simulink model "robo"  (R2024b)
settings: Solver=ode45  StartTime=0.0  StopTime=inf  FixedStep=0.050  RelTol=1e-3
model workspace (MAT data in the model file):
  Sig = Simulink.Signal
  Sig.Dimensions = -1
  Sig.DimensionsMode = 'auto'
  Sig.Complexity = 'auto'
  Sig.SampleTime = -1
  Sig.SamplingMode = 'auto'
  Sig.DataType = 'auto'
  Var = 0
libraries: fuzblock x2
settings Model: PauseTimes=7  Creator=user  LastModifiedBy=manav
settings SolverCC: AlgebraicLoopSolver=TrustRegion
settings DataIOCC: LimitDataPoints=on  SaveFormat=Array  ReturnWorkspaceOutputs=off
settings OptimizationCC: BlockReduction=off  BooleanDataType=off  LifeSpan=inf
settings DebuggingCC: SaveWithParameterizedLinksMsg=none  UnderspecifiedInitializationDetection=Classic  MergeDetectMultiDrivingBlocksExec=none  SignalResolutionControl=TryResolveAllWithWarning  UnconnectedInputMsg=warning  UnconnectedOutputMsg=warning  UnconnectedLineMsg=warning  SFUnexpectedBacktrackingDiag=warning  SFNoUnconditionalDefaultTransitionDiag=warning  SFExecutionAtInitializationDiag=none  ArithmeticOperatorsInVariantConditions=warning
settings HardwareCC: ProdBitPerPointer=32  ProdBitPerSizeT=32  ProdBitPerPtrDiffT=32  ProdLargestAtomicFloat=None  ProdIntDivRoundTo=Undefined  ProdEndianess=Unspecified  ProdWordSize=32  ProdHWDeviceType=32-bit Generic  TargetUnknown=on
settings ModelReferenceCC: EnableRefExpFcnMdlSchedulingChecks=on  PropagateSignalLabelsOutOfModel=off
settings SFSimCC: SimUseLocalCustomCode=off  CustomCodeUndefinedFunction=UseInterfaceOnly
settings RTWCC: RTWUseLocalCustomCode=off  GPUComputeCapability=3.5
settings CodeAppCC: StateflowObjectComments=on
settings GRTTargetCC: TargetLangStandard=C89/C90 (ANSI)
settings ConfigComp: CovMetricSettings=dw  CovSaveCumulativeToWorkspaceVar=on  CovSaveSingleToWorkspaceVar=on  CovExternalEMLEnable=off  CovSFcnEnable=off

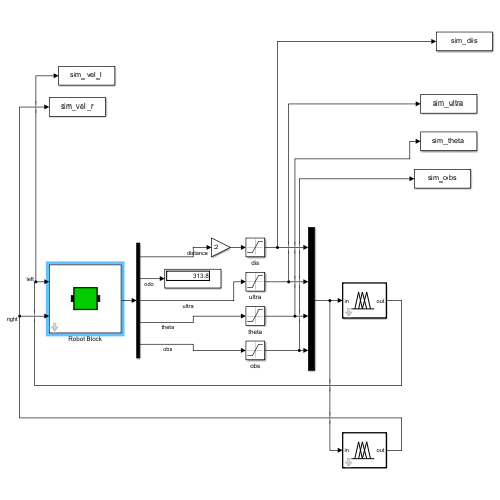
[thumbnail: Simulink's stored preview of the top-level diagram]
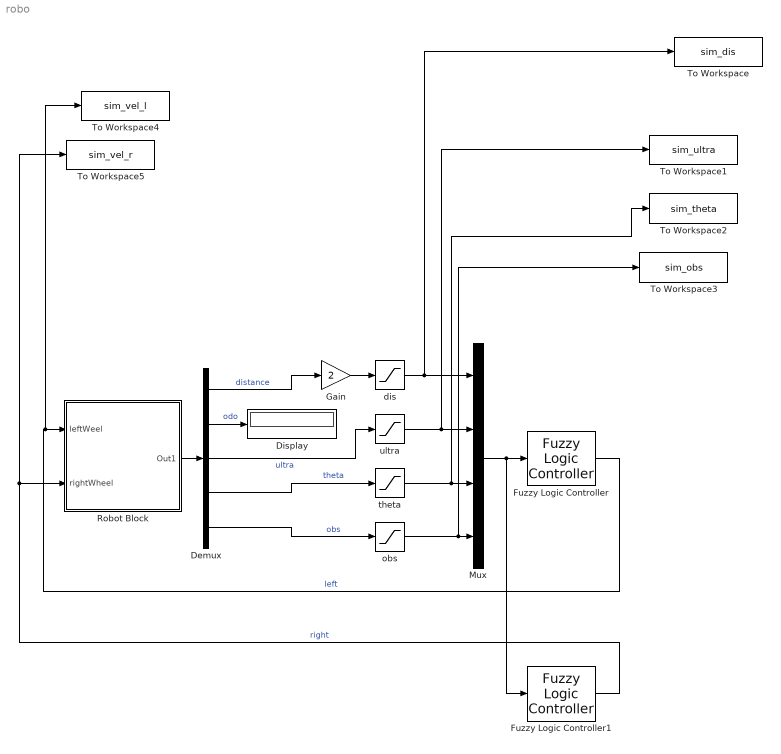
== system robo ==
  Demux : Demux  Outputs=5
  Display : Display
  Fuzzy Logic Controller : fuzblock/Fuzzy Logic  Controller  FIS='anfis_l.fis'  OutputSampleNumber=101  DataType=double  FuzzifiedInputs=off  RuleFiringStrengths=off  RuleOutputs=off  AggregatedOutputs=off  SimulateUsing=Interpreted execution  OutOfRangeInputValueMessage=warning  NoRuleFiredMessage=warning  EmptyOutputFuzzySetMessage=warning
  Fuzzy Logic Controller1 : fuzblock/Fuzzy Logic  Controller  FIS='anfis_r.fis'  OutputSampleNumber=101  DataType=double  FuzzifiedInputs=off  RuleFiringStrengths=off  RuleOutputs=off  AggregatedOutputs=off  SimulateUsing=Interpreted execution  OutOfRangeInputValueMessage=warning  NoRuleFiredMessage=warning  EmptyOutputFuzzySetMessage=warning
  Gain : Gain  Gain=2
  Mux : Mux
  Robot Block : Subsystem  mask(Two-wheel Mobile Robot Model){stID=8199607, modeVal=off, initAngle=1.696, simStep=0.050, Xpos=3.4, Ypos=5.8, isDemo=off}
      mask prompts: stID "Please Enter your UOW student number"; modeVal "Velocity Measurement Mode, select this to disable animations and to allow for the measurement of the velocity of the robot"; initAngle "Set the starting angle (Radians)"; simStep "Override Simulation Step (Defualt is 0.01)"; Xpos "(X,Y)"
      mask help:
      | Robot: Two-wheel robot is driven by two parallel wheels; the speed of each wheel could be set separately
      | Target: target is a single moving point in 2D space
      | Obstacle: obstacle is a group of polygons.
      | Block inputs:
      | vl : velocity of left wheel
      | vr : velocity of right wheel
      | Range of vl, vr: [-2, 2]
      | Block outputs:
      | theta: angle between robot facing and target bearing
      | dis: distance between robot and target
      | ob_loc
      | Range of obstacle detection sensor is 2.5
      | ob_loc=-9	No obstacle detected
      | ob_loc=-2.5	obstacle detected on the front left
      | ob_loc=-5	obstacle detected on the side left
      | ob_loc=0	obstacle detected in the middle
      | ob_loc=2.5	obstacle detected on the front right
      | ob_loc=5	obstacle detected on the side right
      | Battery level/Odometer: total remaining energy/Distance Travelled
      | ultrasonic: a logorithmic signal indicating the distance to the obstacle ( ie 0 = out of sight , a larger number = nearer to the obstacle )
      |
      | The system will crash if the robot collides with the obstacle.
      mask init:
      | stObj.stID = stID;
      | stObj.modeVal = modeVal;
      | stObj.simStep = simStep;
      | stObj.initPos = [Xpos Ypos initAngle];
      | stObj.isDemo = isDemo;
      mask Help:
      | Robot: Two-wheel robot is driven by two parallel wheels; the speed of each wheel could be set separately
      | Target: target is a single moving point in 2D space
      | Obstacle: obstacle is a group of polygons.
      | Block inputs:
      | vl : velocity of left wheel
      | vr : velocity of right wheel
      | Range of vl, vr: [-2, 2]
      | Block outputs:
      | theta: angle between robot facing and target bearing
      | dis: distance between robot and target
      | ob_loc
      | Range of obstacle detection sensor is 2.5
      | ob_loc=-9	No obstacle detected
      | ob_loc=-2.5	obstacle detected on the front left
      | ob_loc=-5	obstacle detected on the side left
      | ob_loc=0	obstacle detected in the middle
      | ob_loc=2.5	obstacle detected on the front right
      | ob_loc=5	obstacle detected on the side right
      | Battery level/Odometer: total remaining energy/Distance Travelled
      | ultrasonic: a logorithmic signal indicating the distance to the obstacle ( ie 0 = out of sight , a larger number = nearer to the obstacle )
      | 
      | The system will crash if the robot collides with the obstacle.
      mask Callback simStep:
      | pm = Simulink.Mask.get(gcb);
      | simStep = pm.getParameter('simStep');
      | set_param(gcs,'FixedStep', simStep.Value);
      mask DialogControl Container4 Prompt: Set the initial starting Coordinates and angle
      mask DialogControl Control3 Prompt: Set starting Position , (must be in the red shaded region)
      mask DialogControl Control3 Callback:
      | [out,~,~,~,~] = roboanimate_org([],[],[],'setup',[]);
      | Xpos = out(1);
      | Ypos = out(2);
      | p = Simulink.Mask.get(gcb);
      | p.Parameters(1,5).set('Value',num2str(Xpos));
      | p.Parameters(1,6).set('Value',num2str(Ypos));
      mask DialogControl Control5 Prompt: Initial Position:
      mask DialogControl Container4_copy Prompt: Run a demo
      mask DialogControl Control2 Prompt: Run  demo
      mask DialogControl Control2 Callback:
      | if(get_param(gcs,'SimulationStatus') == 'stopped')
      | 
      | pm = Simulink.Mask.get(gcb);
      | pm.Parameters(1,7).set('Value','on');
      | options = simset('SrcWorkspace','current');
      | try
      | sim(gcs,[],options)
      | pm.Parameters(1,7).set('Value','off');
      | catch
      | pm.Parameters(1,7).set('Value','off');
      | end
      | 
      | end
      mask Display:
      | patch([ -0.5 0.5 0.5 -0.5],[ -0.5 -0.5 0.5 0.5],[1 1 1])
      | 
      | patch([ -0.2 0.2 0.2 -0.2],[ -0.05 -0.05 0.05 0.05],[0 0 0])
      | 
      | patch(1.1*[ -0.15  0.15 0.15 -0.15],1.1*[ -0.15 -0.15 0.15 0.15],[0 0 0])
      | 
      | patch([ -0.15  0.15 0.15 -0.15],[ -0.15 -0.15 0.15 0.15],[0 0.8 0])
  To Workspace : ToWorkspace  VariableName=sim_dis  SaveFormat=Timeseries  SampleTime=-1
  To Workspace1 : ToWorkspace  VariableName=sim_ultra  SaveFormat=Timeseries  SampleTime=-1
  To Workspace2 : ToWorkspace  VariableName=sim_theta  SaveFormat=Timeseries  SampleTime=-1
  To Workspace3 : ToWorkspace  VariableName=sim_obs  SaveFormat=Timeseries  SampleTime=-1
  To Workspace4 : ToWorkspace  VariableName=sim_vel_l  SaveFormat=Timeseries  SampleTime=-1
  To Workspace5 : ToWorkspace  VariableName=sim_vel_r  SaveFormat=Timeseries  SampleTime=-1
  dis : Saturate  UpperLimit=20  LowerLimit=0
  obs : Saturate  UpperLimit=5  LowerLimit=-9
  theta : Saturate  UpperLimit=180  LowerLimit=-180
  ultra : Saturate  UpperLimit=25  LowerLimit=0
  wires:
  Mux/1 -> Fuzzy Logic Controller1/1, Fuzzy Logic Controller/1
  obs/1 -> To Workspace3/1, Mux/4
  Robot Block/1(Out1) -> Demux/1
  Demux/1 -> Gain/1  "distance"
  Demux/2 -> Display/1  "odo"
  Demux/3 -> ultra/1  "ultra"
  Demux/4 -> theta/1  "theta"
  Demux/5 -> obs/1  "obs"
  Fuzzy Logic Controller/1 -> To Workspace4/1, Robot Block/1(leftWeel)  "left"
  Fuzzy Logic Controller1/1 -> To Workspace5/1, Robot Block/2(rightWheel)  "right"
  Gain/1 -> dis/1
  theta/1 -> Mux/3, To Workspace2/1
  ultra/1 -> To Workspace1/1, Mux/2
  dis/1 -> To Workspace/1, Mux/1

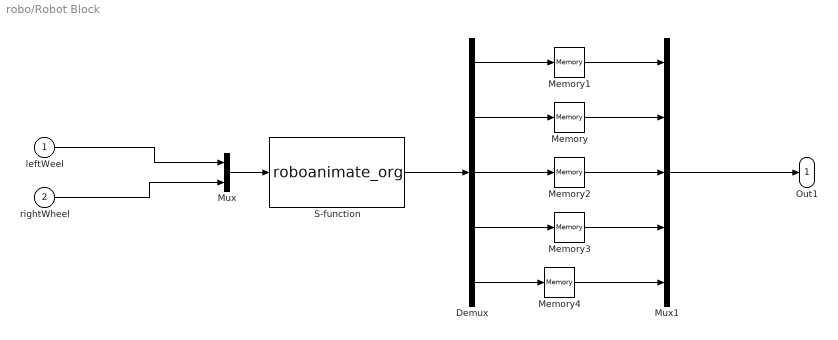
== system robo/Robot Block ==
  leftWeel : Inport
  rightWheel : Inport  Port=2
  Demux : Demux  Outputs=5
  Memory{,2..4} (4 alike) : Memory
  Memory1 : Memory  InitialCondition=1000
  Mux : Mux  Inputs=2
  Mux1 : Mux  Inputs=5
  S-function : S-Function  FunctionName=roboanimate_org  Parameters=stObj  SFunctionDeploymentMode=off  EnableBusSupport=off
  Out1 : Outport
  wires:
  rightWheel/1 -> Mux/2
  leftWeel/1 -> Mux/1
  Mux/1 -> S-function/1
  S-function/1 -> Demux/1
  Memory1/1 -> Mux1/1
  Demux/1 -> Memory1/1
  Memory/1 -> Mux1/2
  Memory2/1 -> Mux1/3
  Demux/3 -> Memory2/1
  Demux/2 -> Memory/1
  Demux/4 -> Memory3/1
  Memory3/1 -> Mux1/4
  Demux/5 -> Memory4/1
  Memory4/1 -> Mux1/5
  Mux1/1 -> Out1/1
